simulink model "dinamicaRRR"  (R2019b)
settings: Solver=FixedStepAuto  StartTime=0.0  StopTime=10  FixedStep=0.001  RelTol=1e-3
InitFcn:
  | init
values from neighbouring files (symbols this model uses):
  g = 9.8    [init.m]
  l1 = 0.5    [init.m]
  l2 = 0.3    [init.m]
  m1 = 4.6    [init.m]
  m2 = 2.3    [init.m]
  m3 = 1.0    (= 1)    [init.m]
settings Model: SimulationMode=accelerator  Creator=vfton  LastModifiedBy=xgge2
settings DebuggingCC: UnconnectedInputMsg=none  UnconnectedOutputMsg=none  UnconnectedLineMsg=none  SFMachineParentedDataDiag=error

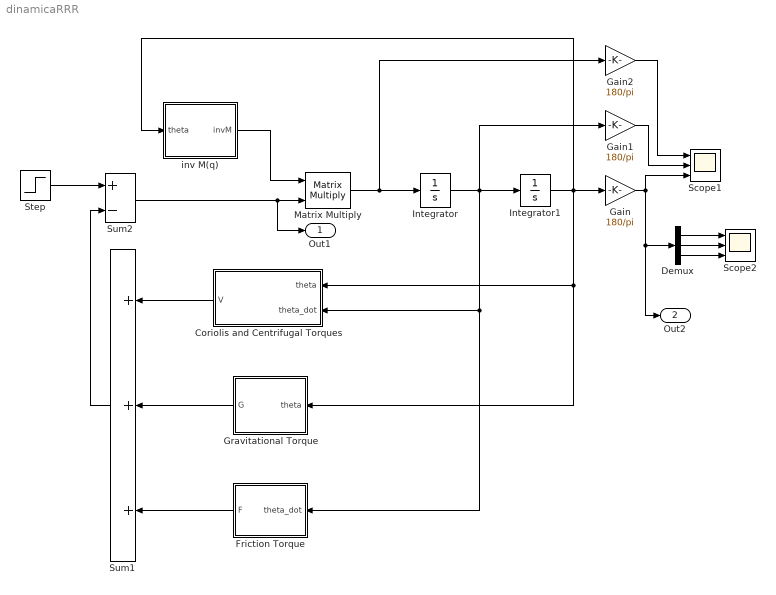
== system dinamicaRRR ==
  "Coriolis and Centrifugal Torques " : MATLAB Function  TreatAsAtomicUnit=on
  Demux : Demux  Outputs=3
  Friction Torque : MATLAB Function  TreatAsAtomicUnit=on
  Gain : Gain  Gain=180/pi
  Gain1 : Gain  Gain=180/pi
  Gain2 : Gain  Gain=180/pi
  Gravitational Torque : MATLAB Function  TreatAsAtomicUnit=on
  Integrator : Integrator  InitialCondition=[0; 0; 0]
  Integrator1 : Integrator  InitialCondition=[-pi/6; pi/6; pi/6]
  Matrix Multiply : Product  Multiplication=Matrix(*)
  Scope1 : Scope  NumInputPorts=3
  Scope2 : Scope  NumInputPorts=3
  Step : Step  Before=[0; 0; 0]  After=[0; 0; 0]  SampleTime=0  VectorParams1D=off
  Sum1 : Sum  Inputs=+++
  Sum2 : Sum  Inputs=+-
  inv M(q) : MATLAB Function  TreatAsAtomicUnit=on
  Out1 : Outport
  Out2 : Outport  Port=2
  wires:
  Step/1 -> Sum2/1
  Sum1/1 -> Sum2/2
  "Coriolis and Centrifugal Torques "/1(V) -> Sum1/1
  Gravitational Torque/1(G) -> Sum1/2
  Friction Torque/1(F) -> Sum1/3
  Sum2/1 -> Out1/1, Matrix Multiply/2
  Matrix Multiply/1 -> Gain2/1, Integrator/1
  Integrator/1 -> Friction Torque/1(theta_dot), "Coriolis and Centrifugal Torques "/2(theta_dot), Gain1/1, Integrator1/1
  Gain2/1 -> Scope1/1
  Gain/1 -> Out2/1, Demux/1, Scope1/3
  Gain1/1 -> Scope1/2
  Integrator1/1 -> inv M(q)/1(theta), Gravitational Torque/1(theta), "Coriolis and Centrifugal Torques "/1(theta), Gain/1
  Demux/1 -> Scope2/1
  Demux/3 -> Scope2/3
  Demux/2 -> Scope2/2
  inv M(q)/1(invM) -> Matrix Multiply/1

== matlab function dinamicaRRR/Gravitational Torque ==
  data: theta input size=[3,1]; G output size=[3,1]; m1 parameter; m2 parameter; l1 parameter; l2 parameter; g parameter; m3 parameter
function G  = fcn(theta, m1, m2, l1, l2, g, m3)
    G = zeros([3,1]);
    G(1) = (m2+m3)*l2*g*cos(theta(1)+theta(2))+(m1+m2+m3)*l1*g*cos(theta(1));
    G(2) = (m2+m3)*l2*g*cos(theta(1)+theta(2));
    G(3) = 0;

== matlab function dinamicaRRR/Coriolis and Centrifugal Torques  ==
  data: theta input size=[3,1]; V output size=[3,1]; theta_dot input size=[3,1]; m2 parameter; l1 parameter; l2 parameter; m3 parameter
function V  = fcn(theta,theta_dot, m2, l1, l2, m3)
    V = zeros([3,1]);
    V(1) = -(m2+m3)*l1*l2*sin(theta(2))*theta_dot(2)^2 - 2*(m2+m3)*l1*l2*sin(theta(2))*theta_dot(1)*theta_dot(2);
    V(2) = (m2+m3)*l1*l2*sin(theta(2))*theta_dot(1)^2;
    V(3) = 0;

== matlab function dinamicaRRR/Friction Torque ==
  data: theta_dot input size=[3,1]; F output size=[3,1]; v parameter
function F = fcn(theta_dot, v)
    F = zeros([3,1]);
    F(1) = v*theta_dot(1);
    F(2) = v*theta_dot(2);
    F(3) = v*theta_dot(3);

== matlab function dinamicaRRR/inv M(q) ==
  data: theta input size=[3,1]; invM output size=[3,3]; m1 parameter; m2 parameter; l1 parameter; l2 parameter; m3 parameter
function invM  = fnc(theta, m1, m2, l1, l2, m3)
    M = zeros([3,3]);
    M(1,1) = 0.1 + (m2+m3)*l2^2 + 2*(m2+m3)*l1*l2*cos(theta(2))+(l1^2)*(m1+m2+m3);
    M(1,2) = 0.1 + (m2+m3)*l2^2 + (m2+m3)*l1*l2*cos(theta(2));
    M(1,3) = 0.1;
    M(2,1) = 0.1 + (m2+m3)*l2^2 + (m2+m3)*l1*l2*cos(theta(2));
    M(2,2) = 0.1 + (m2+m3)*l2^2;
    M(2,3) = 0.1;
    M(3,1) = 0.1;
    M(3,2) = 0.1;
    M(3,3) = 0.1;
    
    invM = inv(M);
